simulink model "Super8"  (Simulink 5.0)
settings: Solver=ode45  StartTime=0.0  StopTime=10.0  RelTol=1e-3
settings Model: Creator=scaife  LastModifiedBy=scaife  ExtModeAutoUpdateStatusClock=off

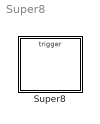
== system Super8 ==
  Super8 : Stateflow chart

== stateflow chart Super8 ==
  state A
    state A1
      state A1a
      (default) -> A1a
    (default) -> A1
  state B
  B -> A1a : E
  (default) -> B
  events: E input EITHER_EDGE_EVENT
